simulink model "Model_TranslationEngine64"  (R2022b)
settings: Solver=FixedStepDiscrete  StartTime=0.0  StopTime=5  RelTol=1e-3  EnableMultiTasking=on
InitFcn:
  | % Initialize model
  | ModelSettings=BTConfig.GetModelSettings();
  | 
  | ModelSettings.Validate();
  | 
  | ModelInit;
  | 
  | 
  | % load library data
  | GainLibrary_data;
  | % Load saved values from partition process
  | CapturedConstMask.LoadMapFromFile(bdroot)
StartFcn:
  | % make sure all the simulated RTC requests are found
  | %RTC_SIM_OBJ.ValidateREQs();
undefined symbols (not defined in the file or in its folder): AA, BPLP, Column, NumHFRefBPF, NumHFRefLPF, NumMusicChannels, Row, VolumeMuteConfig
libraries: TuneVar x925, TOP x490, FeaturePath x111, CapturedConstLib x52
(part 3 of 34)

== system Model_TranslationEngine64/NEAR/Near1p1/DrProc ==
  FeaturePath : FeaturePath/FeaturePath  FeatureName=Dr_  IsGroup=off  GroupNumber=-1  IsModule=off  TriggerInit=[730 -106 845 1]
      settings: SourceProductName=Bose Talaria
  FsEQDr : Subsystem  mask(FsEQ){Config=Config.FsEqDr}
      mask prompts: Config "FsEqConfig"
      mask help:
      | This mask allows the setting of parameters for the FsEQ model.
      | Model parameters are set by a class instance in the base workspace.
      |
      | See 'Help' for details.
      mask init:
      | blkh=gcbh;
      | Config=BTConfig.Assert(blkh,Config);
      | 
      | Config.Validate();
      | Config.DoMaskInit(blkh);
      mask Help:
      | Defining model parameters:
      | The model parameters are set by the conents of an instance of FsEQClass.m.
      | 
      | To set model parameters:
      | 1-Create an instance of FsEQClass.m in the base workspace.
      | 2-In the model mask, set the 'Class instance' parameter to the name of the class instance in the base workspace.
      mask DialogControl ClassContainer Prompt: Name of class instance containing parameter settings
  HrEQDr : Subsystem  mask(HrEQ){Config=Config.HrEqDr}
      mask prompts: Config "HrEqConfig"
      mask help:
      | This mask allows the setting of parameters for the HrEQ model.
      | Model parameters are set by a class instance in the base workspace.
      |
      | See 'Help' for details.
      mask init:
      | blkh=gcbh;
      | Config=BTConfig.Assert(blkh,Config);
      | 
      | Config.Validate();
      | Config.DoMaskInit(blkh);
      mask Help:
      | Defining model parameters:
      | The model parameters are set by the conents of an instance of HrEQClass.m.
      | 
      | To set model parameters:
      | 1-Create an instance of HrEQClass.m in the base workspace.
      | 2-In the model mask, set the 'Class instance' parameter to the name of the class instance in the base workspace.
  RouterDr : Subsystem  mask(Bose Router){nInRouterMask=Config.NearRouterNumIn, nOutRouterMask=Config.NearRouterNumOut, outputMapDefaultRouterMask=Config.NearRouterMap}
      mask prompts: nInRouterMask "Number of input channels"; nOutRouterMask "Number of output channels"; outputMapDefaultRouterMask "Router output channel indices"
      mask help: This block allows the user to route X input channels to Y output channels. Enter a value of 0 to "zero out" the specific channel
      mask init:
      | blkh = gcbh;
      | % Copy discrete mask parameters into a classdef object
      | InnerLinkConfig = RouterConfig;
      | InnerLinkConfig.NumIn = nInRouterMask;
      | InnerLinkConfig.NumOut = nOutRouterMask;
      | InnerLinkConfig.DefaultOutputMap = outputMapDefaultRouterMask;
      mask Display: image('routerIcon.png');
  Upmixer1p1Dr : Subsystem  mask{Config=Config.Upmixer1p1Dr}
      mask prompts: Config "Upmixer1p1Config"
      mask init:
      | blkh=gcbh;
      | Config=BTConfig.Assert(blkh,Config);
      | % frontPeripheralChannelCount     = upmixer.front_peripheral_channel_count;
      | % headrest_count                  = upmixer.headrest_count;
      | % channels_per_headrest           = upmixer.channels_per_headrest;
      | Config.Validate();
      | Config.DoMaskInit(blkh);

== system Model_TranslationEngine64/NEAR/Near1p1/FrProc ==
  Subsystem : Subsystem

== system Model_TranslationEngine64/NEAR/Near1p1/LocRamper ==
  TuneTOP : Subsystem  mask(Talaria Trivial Tune TOP){TriggerInit=[-300 49 -55 141], TopName=RampDbPerSample, TuneName=RampDbPerSample, DataTypeOut=single, MaskValue=Config.DefaultRampDbPerSample, TunabilityNumber=1, MinValue=[], MaxValue=[], BankNumber=0, PreOverlay=false, PostOverlay=false, UseSameName=on}
      mask prompts: TriggerInit "Hidden: MoveFcn redraw"; TopName "Name:"; TuneName "Name of TuneVar:"; DataTypeOut "Data type:"; MaskValue "Default Value:"; TunabilityNumber "Tunability:"; MinValue "Min Value:"; MaxValue "Max Value:"; BankNumber "Target memory bank number:"; PreOverlay "Requires pre-overlay action:"; PostOverlay "Requires post-overlay action:"; UseSameName "Use same name for tune variable and TOP"
      mask help: The TuneTOP block encapsultes a Target Overlay Parameter, a Tune Variable, and a Trivial Translation between them.
      mask init:
      | [ok,activeTopPath,activeTunePath] = TuneTOP_Mask.Init(gcbh);
      settings: MoveFcn=TuneTOP_Mask.CB_TriggerInit(gcbh);
      mask Callback TriggerInit: TuneTOP_Mask.CB_TriggerInit(gcbh);
      mask TypeOptions TopName: TOP/TopName
      mask TypeOptions TuneName: Tune Variable/TuneName
      mask TypeOptions DataTypeOut: TOP/DataTypeOut
      mask TypeOptions MaskValue: Tune Variable/MaskValue
      mask TypeOptions TunabilityNumber: Tune Variable/TunabilityNumber
      mask Callback TunabilityNumber: TuneVarMask.CB_TunabilityNumber(gcbh);
      mask TypeOptions MinValue: Tune Variable/MinValue
      mask TypeOptions MaxValue: Tune Variable/MaxValue
      mask TypeOptions BankNumber: TOP/BankNumber
      mask TypeOptions PreOverlay: TOP/PreOverlay
      mask TypeOptions PostOverlay: TOP/PostOverlay
      mask Callback UseSameName: TuneTOP_Mask.CB_UseSameName(gcbh);
      mask DialogControl toolPanel Prompt: Tuning Tool Hints
      mask DialogControl DescriptionGroup Prompt: Description
      mask DialogControl EditDescription Prompt: Edit Description
      mask DialogControl EditDescription Callback: TuneTOP_Mask.CB_EditDescription(gcbh);
      mask DialogControl TunabilityText Prompt: Easy: Changes nearly every tuning.
      mask DialogControl AdvancedPanel Prompt: Advanced
      mask DialogControl ConvertToFullTranslation Prompt: Irreversible conversion to full translation
      mask DialogControl ConvertToFullTranslation Callback: TuneTOP_Mask.CB_ConvertToFullTranslation(gcbh);
      mask DialogControl ErrorContainer Prompt: Error Messages
      mask Display:
      | % retrieve icon definition
      | [path,w,h] = TuneTOP_Mask.Icon();
      | 
      | % retrieve the block's pixel size
      | pos = get(gcbh,'position');
      | bw = pos(3) - pos(1);
      | bh = pos(4) - pos(2);
      | 
      | % draw centered icon
      | xAdj = bw/2 - w/2 + 5;
      | yAdj = bh/2 - h/2 + 4;
      | for i=1:length(path)
      | 	patch(path(i).x+xAdj, path(i).y+yAdj, path(i).rgb);
      | end
      | 
      | % show the top name or an X
      | if (exist('ok','var') && ok)
      | 	text(bw*0.5, bh*0.2, activeTopPath, 'horizontalAlignment', 'center');
      | 	patch(0,0,[1 1 1]);
      | 	patch(bw,bh,[1 1 1]);
      | else
      | 	tx=bw*0.03;
      | 	ty=bh*0.03;
      | 	patch([0 tx bw bw-tx], [ty 0 bh-ty bh], [1 0 0]);
      | 	patch([0 bw-tx bw tx], [bh-ty 0 ty bh], [1 0 0]);
      | end

== system Model_TranslationEngine64/NEAR/Near1p1/NearBandSplit ==
  HighpassFilter : Subsystem

== system Model_TranslationEngine64/NEAR/Near1p1/VolumeMute ==
  AnnouncementLevelDetector : Subsystem  mask(Level Detector for AudioPilot, Dyanmic EQ, Fan and Boost-on-Demand){vm=VolumeMuteConfig, DefaultFlag=off, Config=Config.AnnouncementLevelDetector}
      mask prompts: vm "Vm Class Instance"; DefaultFlag "Use Default Configuration Only"; Config "AnnouncementLevelDetectorConfig"
      mask help: This block performs level detection, separately and independently, for various features. These include AudioPilot, Dynamic Equalization, Amplifier Fan Control, and Boost on Demand. The block is designed to accept as input the entertainment audio channels before volume control was applied. The volume setting, in linear, forms a different input.
      mask init:
      | blkh=gcbh;
      | Config=BTConfig.Assert(blkh,Config);
      | % if DefaultFlag
      | %     LD = struct();
      | % end
      | %[LD, SampleRate, FrameRate, MaxMusicDelay] ...
      | %    = AnnouncementLevelDetectionMask.Initialize(gcbh,LD,vm);
      | Config.Validate();
      | Config.DoMaskInit(blkh);
      mask Callback DefaultFlag: % AnnouncementLevelDetectionMask.DefaultFlagCallBack(gcbh);
  VolMuteCh1 : Subsystem
  VolMuteCh2 : Subsystem
  VolMuteCh3 : Subsystem
  VolMuteCh4 : Subsystem

== system Model_TranslationEngine64/PostProcess/PostProcess/Limiter ==
  Limiter : Subsystem  mask(Blocklib Limiter){Config=Config.Limiter, FeatureName=Limiter}
      mask prompts: Config "LimiterConfig"; FeatureName "Feature path name:"
      mask init:
      | blkh=gcbh;
      | Config=BTConfig.Assert(blkh,Config);
      | 
      | Config.Validate();
      | BTConfig.InitSetFeatureIfPresent(blkh,'FeatureName');
      mask Callback Config: BTConfig.CallbackHideIfPresent(gcbh,{'FeatureName'});
      mask TypeOptions FeatureName: FeaturePath/FeatureName
      mask Display:
      | [path,w,h] = IconLimiterMask();
      | 
      | % work in pixels since the icon does not scale
      | pos = get(gcbh,'position');
      | bw = pos(3) - pos(1);
      | bh = pos(4) - pos(2);
      | 
      | % Draw centered icon
      | xAdj = bw/2 - w/2;
      | yAdj = bh/2 - h/2 + 4;
      | for i=1:length(path)
      |     if (path(i).rgb(1) >= 0)
      |         patch(path(i).x+xAdj, path(i).y+yAdj, path(i).rgb);
      |     end
      |     if (path(i).stroke(1) >= 0)
      |         plot(path(i).x+xAdj, path(i).y+yAdj);
      |     end
      | end
      | 
      | % Display some text
      | text(bw/2, 4,FeatureName, ...
      |     'horizontalAlignment','center', ...
      |     'VerticalAlignment','bottom');

== system Model_TranslationEngine64/PostProcess/PostProcess/Mute ==
  Mute : Subsystem  mask(Blocklib Mute){Config=Config.Mute, FeatureName=Mute}
      mask prompts: Config "MuteConfig"; FeatureName "Feature path name:"
      mask help: This block offers a simple mute feature using rgainy block. Set initial mute state for system cold start and a feature path name as desired. There are no tunable components, but runtime control is included.
      mask init:
      | blkh=gcbh;
      | Config=BTConfig.Assert(blkh,Config);
      | BTConfig.InitSetFeatureIfPresent(blkh,'FeatureName');
      | Config.Validate();
      mask Help:
      | This block offers a simple mute feature using rgainy block. The initial mute status of the block can be set through the mask.
      | 
      | RTC CONTROL:
      | Run time control is available to dynamically mute the audio. The mute status can be provided ('1' to mute audio), along with a ramp time and rate (rate gets precedence).
      | RTC_SIM_OBJ.AddREQ( 'MuteSet', 0.6, [0005,  <mute_status>, <ramp_db_per_second>, <ramp_time>]);
      | E.g., RTC_SIM_OBJ.AddREQ( 'MuteSet', 0.7, [0002, 1, 0, 50]);
      mask Callback Config: BTConfig.CallbackHideIfPresent(gcbh,{'FeatureName'});
      mask TypeOptions FeatureName: MuteControl/FeatureName
      mask Display:
      | [path,w,h] = IconMuteMask();
      | 
      | % work in pixels since the icon does not scale
      | pos = get(gcbh,'position');
      | bw = pos(3) - pos(1);
      | bh = pos(4) - pos(2);
      | 
      | % Draw centered icon
      | xAdj = bw/2 - w/2;
      | yAdj = bh/2 - h/2;
      | for i=1:length(path)
      |     if (path(i).rgb(1) >= 0)
      |         patch(path(i).x+xAdj, path(i).y+yAdj, path(i).rgb);
      |     end
      |     if (path(i).stroke(1) >= 0)
      |         plot(path(i).x+xAdj, path(i).y+yAdj);
      |     end
      | end
      | 
      | % Display some text
      | text(bw/2, 2,FeatureName, ...
      |     'horizontalAlignment','center', ...
      |     'VerticalAlignment','bottom');

== system Model_TranslationEngine64/PostProcess/PostProcess/PostLimiterEQ ==
  PoolIirTunableWithReset : Subsystem  mask(Bose Pool IIR Tunable){FeatureName=PostLimiterEq, Config=Config.PostLimiterEq}
      mask prompts: FeatureName "Filter name/purpose"; Config "PoolIirTunableWithResetConfig"
      mask help:
      | Pool IIR Tunable is a configurable multi-channel IIR filter that supports one or more channels. This block offers flexibility of tuning the number of stages and coefficients. Different filter coefficients and number of stages (biquads) can be used for each channel filter. The Pool IIR Tunable block supports different implementations, which could be configured at build-time:
      |
      | (i)   Generic: IIR filter code not optimized for any processor
      | (ii)  SharcCore: IIR filters executing on core (uses pooliir.asm CRL)
      | (iii) SharcGulAccel: IIR filters executing on IIR hardware accelerator, offloading MIPS usage from core
      | (iv) SharcGxpAccel: IIR filters take advantage of additional accelerators available on GXP processor
      | (v)  Hexagon: TBD
      |
      | NOTE: When using Pool IIR for Sharc-plus based processors, the codeWorkMemory buffer and input buffer should always be mapped to L1 memory to optimize MIPS utilization and avoid audio artifacts.
      |
      | For more information, please see 'Help'.
      mask init:
      | blkh=gcbh;
      | Config=BTConfig.Assert(blkh,Config);
      | 
      | BTConfig.InitSetFeatureIfPresent(blkh,'FeatureName');
      | Config.Validate();
      | Config.DoMaskInit(blkh);
      mask Help:
      | <b>Input signals: </b>
      | AudioIn: input channels [frame size x number of channels]
      | ResetTrigger: trigger to reset internal state buffer (usually preferred as a post RMDL step)
      | 
      | <b>Output signals: </b>
      | AudioOut: output channels [frame size x number of channels]
      | 
      | <b>Mask parameters: </b>
      | PoolIirTunableWithResetConfig
      | Filter name/purpose
      mask TypeOptions FeatureName: FeaturePath/FeatureName
      mask Callback Config: BTConfig.CallbackHideIfPresent(gcbh,{'FeatureName'});
      mask Display: DrawPoolIirIcon;

== system Model_TranslationEngine64/PostProcess/PostProcess/Soft Clipper ==
  SoftClipper : Subsystem  mask(Blocklib SoftClipper){Config=Config.SoftClipper, FeatureName=SoftClipper}
      mask prompts: Config "SoftClipperConfig"; FeatureName "Feature path name:"
      mask init:
      | blkh=gcbh;
      | Config=BTConfig.Assert(blkh,Config);
      | 
      | Config.Validate();
      | BTConfig.InitSetFeatureIfPresent(blkh,'FeatureName');
      mask Callback Config: BTConfig.CallbackHideIfPresent(gcbh,{'FeatureName'});
      mask TypeOptions FeatureName: FeaturePath/FeatureName
      mask Display:
      | [path,w,h] = IconSoftclipperMask();
      | 
      | % work in pixels since the icon does not scale
      | pos = get(gcbh,'position');
      | bw = pos(3) - pos(1);
      | bh = pos(4) - pos(2);
      | 
      | % Draw centered icon
      | xAdj = bw/2 - w/2;
      | yAdj = bh/2 - h/2 + 4;
      | for i=1:length(path)
      |     if (path(i).rgb(1) >= 0)
      |         patch(path(i).x+xAdj, path(i).y+yAdj, path(i).rgb);
      |     end
      |     if (path(i).stroke(1) >= 0)
      |         plot(path(i).x+xAdj, path(i).y+yAdj);
      |     end
      | end
      | 
      | % Display some text
      | text(bw/2, 4,FeatureName, ...
      |     'horizontalAlignment','center', ...
      |     'VerticalAlignment','bottom');

== system Model_TranslationEngine64/TestRouter/ASDRouter/InnerLink ==
  AuxChannel_with_MATLAB_function : Subsystem
  FeaturePath : FeaturePath/FeaturePath  FeatureName=ASDRouter  IsGroup=off  GroupNumber=-1  IsModule=off  TriggerInit=[-50 -126 65 -19]
      settings: SourceProductName=Bose Talaria
  MainChannelSystem : Subsystem

== system Model_TranslationEngine64/ModelPreAmp/DecRate/AudioPilot35/Audiopilot_3_5 ==
  ConfigurationRtcInputs : Subsystem
  FeaturePath : FeaturePath/FeaturePath  FeatureName=Audiopilot  IsGroup=off  GroupNumber=-1  IsModule=off  TriggerInit=[1175 264 1290 371]
      settings: SourceProductName=Bose Talaria
  GainApplication : Subsystem  mask(AudioPilot - Loudness Gain Application){NumInputChannels=NumMusicChannels, Config=Config.GainApp}
      mask prompts: NumInputChannels "Number of Input Channels"; Config "GainApplicationConfig"
      mask help: This block implements the necessary compensation to the audio stream for AudioPilot and Dynamic EQ.
      mask init:
      | blkh = gcbh;
      | 
      | Config = BTConfig.Assert(blkh,Config);
      | Config.Validate();
      | 
      | SampleRate = Config.SampleRateHz;
      | FrameSize = Config.FrameSize;
      | oneFrame = ones(FrameSize,1);
      | MaxAlignDelaySamples = Config.MidrangeLpfMaxAlignDelaySamples;
      mask Help:
      | This block implements the necessary compensation to the audio stream for AudioPilot and Dynamic EQ.
      | 
      | Arguments for this block:
      | 
      | Number of Music Channels
      | This is the number of input audio channels to be processed, typically 2 for stereo or 6 for surround.
      | 
      | Build Time Configuration
      | The block can be configured using an object of class, GainApplicationConfig.
      mask DialogControl DTC Prompt: Design Time Configuration
      mask DialogControl BTC Prompt: Build Time Configuration
  GainCalculation : Subsystem  mask(AudioPilot - Gain Calculation){Config=Config.GainCalc}
      mask prompts: Config "GainCalculationConfig"
      mask help: This block implements the gain calculations for AudioPilot and Dynamic EQ.
      mask init:
      | blkh = gcbh;
      | 
      | Config = BTConfig.Assert(blkh,Config);
      | Config.Validate();
      | 
      | SampleRate = Config.SampleRateHz;
      | FrameSize = Config.FrameSize;
      | FrameRate = Config.FrameRateHz;
      | 
      | % Configure RTC responses            
      | GainCalculationMask.ConfigureRtcResponses(blkh,...
      |                 Config.EnableRtcResponse)
      mask Help:
      | This block implements the gain calculations for AudioPilot and Dynamic EQ.
      | 
      | Arguments for this block:
      | 
      | Configuration
      | The block can be configured using an object of class, GainCalculationConfig.
      mask DialogControl BTC Prompt: Build Time Configuration
      mask DialogControl Config Tooltip: The configuration has to be an object of the class, GainCalculationConfig.
  NoiseEstimationVariant : Subsystem  Variant=on  VariantControlMode=label  LabelModeActiveChoice=Regular  PropagateVariantConditions=on

== system Model_TranslationEngine64/ModelPreAmp/DecRate/AudioPilot35/EntertainmentLevelDetection ==
  AudiopilotLevelDetect : Subsystem
  DyneqLevelDetect : Subsystem
  PreProcessing : Subsystem

== system Model_TranslationEngine64/ModelPreAmp/DecRate/AudioPilot35/Volume ==
  FeaturePath : FeaturePath/FeaturePath  FeatureName=VolumeCfg  IsGroup=off  GroupNumber=-1  IsModule=off  TriggerInit=[640 269 755 376]
      settings: SourceProductName=Bose Talaria
  Index2DbTable : Subsystem  mask(Blocklib Index2DbTable){Config=Config}
      mask prompts: Config "Index2DbTableConfig"
      mask help: This block contains overlay tuning data for an index-to-dB lookup table. Provide the maximum number of points in the table as a build-time variable. The TuneVar is variable size, but must define at least two points (i.e. two rows, or four values).
      mask init:
      | blkh=gcbh;
      | Config=BTConfig.Assert(blkh,Config);
      | 
      | Config.Validate();
      mask Help:
      | This block contains overlay tuning data which defines an index-to-dB lookup table.
      | Each row of the tuning data contains an index and a dB value.
      | 
      | Tuning data
      | ---------------
      |    tune index: normalized value between 0 and 1
      |    tune value: dB value such as 0 (aka linear "1") or -100 (aka "very quiet")
      | 
      | Inports
      | ----------
      |    trigger: function call trigger that invokes the lookup from inport index to output dB
      |    index: an 8-bit integer index between [0:255] corresponding to the tuning index range [0:1]
      | 
      | Outport
      | -----------
      |    The resulting dB value looked up in the tuned table by using the inbound index
  TuneVarRampTimeMs : Subsystem  mask(Talaria Trivial Tune TOP){TriggerInit=[825 324 910 356], TopName=RampTime, TuneName=RampTime, DataTypeOut=single, MaskValue=100, TunabilityNumber=1, MinValue=[], MaxValue=[], BankNumber=0, PreOverlay=false, PostOverlay=false, UseSameName=on}
      mask prompts: TriggerInit "Hidden: MoveFcn redraw"; TopName "Name:"; TuneName "Name of TuneVar:"; DataTypeOut "Data type:"; MaskValue "Default Value:"; TunabilityNumber "Tunability:"; MinValue "Min Value:"; MaxValue "Max Value:"; BankNumber "Target memory bank number:"; PreOverlay "Requires pre-overlay action:"; PostOverlay "Requires post-overlay action:"; UseSameName "Use same name for tune variable and TOP"
      mask help: The TuneTOP block encapsultes a Target Overlay Parameter, a Tune Variable, and a Trivial Translation between them.
      mask init:
      | [ok,activeTopPath,activeTunePath] = TuneTOP_Mask.Init(gcbh);
      settings: MoveFcn=TuneTOP_Mask.CB_TriggerInit(gcbh);
      mask Callback TriggerInit: TuneTOP_Mask.CB_TriggerInit(gcbh);
      mask TypeOptions TopName: TOP/TopName
      mask TypeOptions TuneName: Tune Variable/TuneName
      mask TypeOptions DataTypeOut: TOP/DataTypeOut
      mask TypeOptions MaskValue: Tune Variable/MaskValue
      mask TypeOptions TunabilityNumber: Tune Variable/TunabilityNumber
      mask Callback TunabilityNumber: TuneVarMask.CB_TunabilityNumber(gcbh);
      mask TypeOptions MinValue: Tune Variable/MinValue
      mask TypeOptions MaxValue: Tune Variable/MaxValue
      mask TypeOptions BankNumber: TOP/BankNumber
      mask TypeOptions PreOverlay: TOP/PreOverlay
      mask TypeOptions PostOverlay: TOP/PostOverlay
      mask Callback UseSameName: TuneTOP_Mask.CB_UseSameName(gcbh);
      mask DialogControl toolPanel Prompt: Tuning Tool Hints
      mask DialogControl DescriptionGroup Prompt: Description
      mask DialogControl EditDescription Prompt: Edit Description
      mask DialogControl EditDescription Callback: TuneTOP_Mask.CB_EditDescription(gcbh);
      mask DialogControl TunabilityText Prompt: Easy: Changes nearly every tuning.
      mask DialogControl AdvancedPanel Prompt: Advanced
      mask DialogControl ConvertToFullTranslation Prompt: Irreversible conversion to full translation
      mask DialogControl ConvertToFullTranslation Callback: TuneTOP_Mask.CB_ConvertToFullTranslation(gcbh);
      mask DialogControl ErrorContainer Prompt: Error Messages
      mask Display:
      | % retrieve icon definition
      | [path,w,h] = TuneTOP_Mask.Icon();
      | 
      | % retrieve the block's pixel size
      | pos = get(gcbh,'position');
      | bw = pos(3) - pos(1);
      | bh = pos(4) - pos(2);
      | 
      | % draw centered icon
      | xAdj = bw/2 - w/2 + 5;
      | yAdj = bh/2 - h/2 + 4;
      | for i=1:length(path)
      | 	patch(path(i).x+xAdj, path(i).y+yAdj, path(i).rgb);
      | end
      | 
      | % show the top name or an X
      | if (exist('ok','var') && ok)
      | 	text(bw*0.5, bh*0.2, activeTopPath, 'horizontalAlignment', 'center');
      | 	patch(0,0,[1 1 1]);
      | 	patch(bw,bh,[1 1 1]);
      | else
      | 	tx=bw*0.03;
      | 	ty=bh*0.03;
      | 	patch([0 tx bw bw-tx], [ty 0 bh-ty bh], [1 0 0]);
      | 	patch([0 bw-tx bw tx], [bh-ty 0 ty bh], [1 0 0]);
      | end

== system Model_TranslationEngine64/ModelPreAmp/DecRate/Medusa5H1/Balance ==
  Balance : Subsystem  mask(Blocklib Balance){FeatureName=Balance_Cfg, Config=Config.Balance_Cfg}
      mask prompts: FeatureName "Feature path name:"; Config "BalanceConfig"
      mask help:
      | This Balance block allows for runtime control of balancing between left and right speakers/content. Based on a gain index which comes in through a control message, channel gains for 4 different content types are computed: Left, Right, Center, and Mono.
      |
      | For the Channel to Ramper Map, enter any of the following values:
      | 1 - left channel
      | 2 - right channel
      | 3 - center channel
      | 4 - mono channel
      | -1 - unused channel (will esentially be muted)
      |
      | Enable Silent Extreme if the desired outcome when accepting an index of 0 (hard left) or 255 (hard right) should completely mute the opposing channel.
      |
      | If Silent Extreme Mutes Bass is enabled, then all mono channels will be muted, when Silent Extreme is activated.
      |
      | If this block is being used in conjunction with a stand-alone Sleeping Beauty block, disable the two Silent Extreme options.
      mask init:
      | blkh=gcbh;
      | Config=BTConfig.Assert(blkh,Config);
      | 
      | BTConfig.InitSetFeatureIfPresent(blkh,'FeatureName');
      | Config.Validate();
      | 
      | % Mask init code
      | BalanceMask.Init(blkh);
      | 
      | % Flatten config for MFBs
      | MaskNumRampers = Config.NumRampers;
      | MaskBlockH = blkh;
      | % Set boundary conditions (are these supposed to be BTC?)
      | rampRateBounds = [5,50000];
      | rampTimeBounds = [1,3000];
      mask Help:
      | The Balance block includes runtime control support for adjusting the balance dynamically.
      | - Channels may to be assigned to one of 4 possible rampers. Each channel needs to be assigned to a valid ramper (i.e. 1 - 4, or -1 for unused).
      | - The Index offset determines the index which corresponds to the balance being in the center position (typically 128).
      | - 'Enable silent extreme' mutes the speakers of the group whose gains are being 'cut' when at extreme indices.
      | - 'Disable boost' determines whether a boost is required or not. If selected, the maximum boost will be '1' on the linear scale ('0' in dB), otherwise he boost is calculated based on the curve (typically a maximum of 3 dB).
      | 
      | Control messages can be sent through the RTC block. The block is configured to accept a ramp time or rate (the rate has precedence) and an index which determines the gains for each channel group.
      | E.g., RTC_SIM_OBJ.AddREQ( 'BalanceSet', 0.1, [0001, <balance_index>, <ramp_db_per_second>, <ramp_milliseconds>, <subwoofer_index>, <surround_volume_index>]);
      | E.g., RTC_SIM_OBJ.AddREQ( 'BalanceSet', 0.1, [0001, 255, 0, 50, 128, 192]);
      mask TypeOptions FeatureName: FeaturePath/FeatureName
      mask Callback Config: BTConfig.CallbackHideIfPresent(gcbh,{'FeatureName'});
      mask Display:
      | [path,w,h] = IconBalanceMask();
      | 
      | % work in pixels since the icon does not scale
      | pos = get(gcbh,'position');
      | bw = pos(3) - pos(1);
      | bh = pos(4) - pos(2);
      | 
      | % Draw centered icon
      | xAdj = bw/2 - w/2;
      | yAdj = bh/2 - h/2;
      | for i=1:length(path)
      |     if (path(i).rgb(1) >= 0)
      |         patch(path(i).x+xAdj, path(i).y+yAdj, path(i).rgb);
      |     end
      |     if (path(i).stroke(1) >= 0)
      |         plot(path(i).x+xAdj, path(i).y+yAdj);
      |     end
      | end
      | 
      | % place feature name text
      | text(bw*0.5, 0, [FeatureName '\n\n'], 'horizontalAlignment', 'center');

== system Model_TranslationEngine64/ModelPreAmp/DecRate/Medusa5H1/MedusaHoligram ==
  FeaturePath : FeaturePath/FeaturePath  FeatureName=Medusa  IsGroup=off  GroupNumber=-1  IsModule=off  TriggerInit=[90 69 205 176]
      settings: SourceProductName=Bose Talaria
  Medusa5H1 Part 1 : Subsystem  TreatAsAtomicUnit=on
      settings: RTWSystemCode=Nonreusable function
  Medusa5H1 Part 2 : Subsystem  TreatAsAtomicUnit=on
      settings: RTWSystemCode=Nonreusable function
  Medusa5H1 Part 3 : Subsystem  TreatAsAtomicUnit=on
      settings: RTWSystemCode=Nonreusable function  FunctionWithSeparateData=on
  Medusa5H1 Part 4 : Subsystem  TreatAsAtomicUnit=on  RTWFcnName=MedusaHoligram  RTWFileName=MedusaHoligram
      settings: RTWSystemCode=Nonreusable function  FunctionWithSeparateData=on
  Medusa5H1 Part 6 : Subsystem  TreatAsAtomicUnit=on
      settings: RTWSystemCode=Nonreusable function  FunctionWithSeparateData=on

== system Model_TranslationEngine64/ModelPreAmp/DecRate/Medusa5H1/MedusaPostHoligram ==
  MedusaPostHoligram : Subsystem  TreatAsAtomicUnit=on  mask{config=Config.MedusaConfig}
      mask prompts: config "Config struct name:"
      settings: RTWSystemCode=Nonreusable function  RTWFcnNameOpts=Use subsystem name  RTWFileNameOpts=Use subsystem name  FunctionWithSeparateData=on

== system Model_TranslationEngine64/ModelPreAmp/DecRate/Medusa5H1/NearWiggleFilters ==
  NEAR : Subsystem  Variant=on  VariantControl=Variant1

== system Model_TranslationEngine64/ModelPreAmp/DecRate/Medusa5H1/SleepingBeauty ==
  SleepingBeauty : Subsystem  Variant=on  VariantControl=Choice

== system Model_TranslationEngine64/ModelPreAmp/DecRate/Medusa5H1/VLS ==
  Crosstalk Cancellation : Subsystem  mask{configStruct=configStruct.XtalkCancellationConfig}
      mask prompts: configStruct "Config struct name:"
      mask init:
      | IIR = configStruct.IIR;
      mask Display:
      | port_label('input', 1, sprintf('Le_D, Re_D,\nLe_P, Re_P'));
      | port_label('output', 1, 'SpkrOut');
  FeaturePath : FeaturePath/FeaturePath  FeatureName=VLS  IsGroup=off  GroupNumber=-1  IsModule=off  TriggerInit=[1295 -226 1410 -119]
      settings: SourceProductName=Bose Talaria
  VLS Generation - D : Subsystem  mask{configStruct=configStruct.VLSGenDConfig, FeatureName=GenerationDrv}
      mask prompts: configStruct "Config struct name:"; FeatureName "Feature path name:"
      mask init:
      | % Get block parameters from configStruct
      | variantFIR = configStruct.variantFIR;
      | frameSize = configStruct.frameSize;
      | numFilters = configStruct.numFilters;
      | maxTotalFirLength = configStruct.maxTotalFirLength;
      | 
      | % Get block default values
      | firCoeffsDefault = configStruct.firCoeffsDefault;
      | firLengthsDefault = configStruct.firLengthsDefault;
      | 
      | % Set implementation type for FIR
      | % firBlockPath = MaskUtil.SubBlockName(gcbh, 'FIR');
      | % firBlockHandle = getSimulinkBlockHandle(firBlockPath);
      | % if -1 ~= firBlockHandle
      | %     set_param(firBlockHandle, 'variantSelect', variantFIR);
      | %     if variantFIR == 1 % Set two extras block params for Accel implementation
      | %         set_param(firBlockHandle, 'numIn', num2str(4));
      | %         set_param(firBlockHandle, 'frameSize', num2str(frameSize));
      | %     end
      | % end
      mask TypeOptions FeatureName: FeaturePath/FeatureName
  VLS Generation - P : Subsystem  mask{configStruct=configStruct.VLSGenPConfig, FeatureName=GenerationPax}
      mask prompts: configStruct "Config struct name:"; FeatureName "Feature path name:"
      mask init: same as Model_TranslationEngine64/ModelPreAmp/DecRate/Medusa5H1/VLS/VLS Generation - D
      mask TypeOptions FeatureName: FeaturePath/FeatureName

== system Model_TranslationEngine64/ModelPreAmp/PreAmpPart1/Bass/TuneVarOffset ==
  TOP : TOP/TOP  TriggerInit=[440 20 585 80]  TopName=Offset  DataTypeOut=single  BankNumber=BankNumber  PreOverlay=PreOverlay  PostOverlay=PostOverlay  Role=Automatic
      settings: SourceProductName=Bose Talaria
  TrivialTranslation : TuneVar/TrivialTranslation  TriggerInit=[300 28 350 72]
      settings: SourceProductName=Bose Talaria
  Tune Variable : TuneVar/TuneVar  TuneName=Offset  SpecifyMaxSize=off  VariableDim=1 (Row)  MaxSize=[1 1]  TunabilityNumber=1  MinValue=MinValue  MaxValue=MaxValue  TriggerInit=[20 25 190 75]  MaskValue=MaskValue
      settings: SourceProductName=Bose Talaria
  wires:
  Tune Variable/1 -> TrivialTranslation/1  "Offset"
  TrivialTranslation/1 -> TOP/1

== system Model_TranslationEngine64/ModelPreAmp/PreAmpPart1/Bass/TuneVarRampTime ==
  TOP : TOP/TOP  TriggerInit=[440 20 585 80]  TopName=ramptime  DataTypeOut=single  BankNumber=BankNumber  PreOverlay=PreOverlay  PostOverlay=PostOverlay  Role=Automatic
      settings: SourceProductName=Bose Talaria
  TrivialTranslation : TuneVar/TrivialTranslation  TriggerInit=[300 28 350 72]
      settings: SourceProductName=Bose Talaria
  Tune Variable : TuneVar/TuneVar  TuneName=ramptime  SpecifyMaxSize=off  VariableDim=1 (Row)  MaxSize=[1 1]  TunabilityNumber=1  MinValue=MinValue  MaxValue=MaxValue  TriggerInit=[20 25 190 75]  MaskValue=MaskValue
      settings: SourceProductName=Bose Talaria
  wires:
  Tune Variable/1 -> TrivialTranslation/1  "ramptime"
  TrivialTranslation/1 -> TOP/1

== system Model_TranslationEngine64/ModelPreAmp/PreAmpPart1/Bass/TuneVarScale ==
  TOP : TOP/TOP  TriggerInit=[440 20 585 80]  TopName=Scale  DataTypeOut=single  BankNumber=BankNumber  PreOverlay=PreOverlay  PostOverlay=PostOverlay  Role=Automatic
      settings: SourceProductName=Bose Talaria
  TrivialTranslation : TuneVar/TrivialTranslation  TriggerInit=[300 28 350 72]
      settings: SourceProductName=Bose Talaria
  Tune Variable : TuneVar/TuneVar  TuneName=Scale  SpecifyMaxSize=off  VariableDim=1 (Row)  MaxSize=[1 1]  TunabilityNumber=1  MinValue=MinValue  MaxValue=MaxValue  TriggerInit=[20 25 190 75]  MaskValue=MaskValue
      settings: SourceProductName=Bose Talaria
  wires:
  Tune Variable/1 -> TrivialTranslation/1  "Scale"
  TrivialTranslation/1 -> TOP/1

== system Model_TranslationEngine64/ModelPreAmp/PreAmpPart1/Midrange/TuneVarOffset ==
  TOP : TOP/TOP  TriggerInit=[440 20 585 80]  TopName=Offset  DataTypeOut=single  BankNumber=BankNumber  PreOverlay=PreOverlay  PostOverlay=PostOverlay  Role=Automatic
      settings: SourceProductName=Bose Talaria
  TrivialTranslation : TuneVar/TrivialTranslation  TriggerInit=[300 28 350 72]
      settings: SourceProductName=Bose Talaria
  Tune Variable : TuneVar/TuneVar  TuneName=Offset  SpecifyMaxSize=off  VariableDim=1 (Row)  MaxSize=[1 1]  TunabilityNumber=1  MinValue=MinValue  MaxValue=MaxValue  TriggerInit=[20 25 190 75]  MaskValue=MaskValue
      settings: SourceProductName=Bose Talaria
  wires:
  Tune Variable/1 -> TrivialTranslation/1  "Offset"
  TrivialTranslation/1 -> TOP/1

== system Model_TranslationEngine64/ModelPreAmp/PreAmpPart1/Midrange/TuneVarRampTime ==
  TOP : TOP/TOP  TriggerInit=[440 20 585 80]  TopName=RampTime  DataTypeOut=single  BankNumber=BankNumber  PreOverlay=PreOverlay  PostOverlay=PostOverlay  Role=Automatic
      settings: SourceProductName=Bose Talaria
  TrivialTranslation : TuneVar/TrivialTranslation  TriggerInit=[300 28 350 72]
      settings: SourceProductName=Bose Talaria
  Tune Variable : TuneVar/TuneVar  TuneName=RampTime  SpecifyMaxSize=off  VariableDim=1 (Row)  MaxSize=[1 1]  TunabilityNumber=1  MinValue=MinValue  MaxValue=MaxValue  TriggerInit=[20 25 190 75]  MaskValue=MaskValue
      settings: SourceProductName=Bose Talaria
  wires:
  Tune Variable/1 -> TrivialTranslation/1  "RampTime"
  TrivialTranslation/1 -> TOP/1

== system Model_TranslationEngine64/ModelPreAmp/PreAmpPart1/Midrange/TuneVarScale ==
  TOP : TOP/TOP  TriggerInit=[440 20 585 80]  TopName=Scale  DataTypeOut=single  BankNumber=BankNumber  PreOverlay=PreOverlay  PostOverlay=PostOverlay  Role=Automatic
      settings: SourceProductName=Bose Talaria
  TrivialTranslation : TuneVar/TrivialTranslation  TriggerInit=[300 28 350 72]
      settings: SourceProductName=Bose Talaria
  Tune Variable : TuneVar/TuneVar  TuneName=Scale  SpecifyMaxSize=off  VariableDim=1 (Row)  MaxSize=[1 1]  TunabilityNumber=1  MinValue=MinValue  MaxValue=MaxValue  TriggerInit=[20 25 190 75]  MaskValue=MaskValue
      settings: SourceProductName=Bose Talaria
  wires:
  Tune Variable/1 -> TrivialTranslation/1  "Scale"
  TrivialTranslation/1 -> TOP/1

== system Model_TranslationEngine64/ModelPreAmp/PreAmpPart1/NEARPreAmp/FixedAttenuator ==
  "Attenuation " : Subsystem

== system Model_TranslationEngine64/ModelPreAmp/PreAmpPart1/NEARPreAmp/Monoizer ==
  Monoizer : Subsystem  Variant=on  VariantControl=Choice

== system Model_TranslationEngine64/ModelPreAmp/PreAmpPart1/NEARPreAmp/MusicLimiter ==
  annPredTuneTOP : Subsystem
  limiter : Subsystem
      mask DialogControl Container3 Prompt: Parameter Set
      mask Display:
      | [path,w,h] = IconLimiterMask();
      | 
      | % work in pixels since the icon does not scale
      | pos = get(gcbh,'position');
      | bw = pos(3) - pos(1);
      | bh = pos(4) - pos(2);
      | 
      | % Draw centered icon
      | xAdj = bw/2 - w/2;
      | yAdj = bh/2 - h/2 + 4;
      | for i=1:length(path)
      |     if (path(i).rgb(1) >= 0)
      |         patch(path(i).x+xAdj, path(i).y+yAdj, path(i).rgb);
      |     end
      |     if (path(i).stroke(1) >= 0)
      |         plot(path(i).x+xAdj, path(i).y+yAdj);
      |     end
      | end
      | 
      | % Anchor the corners of the coordinate system
      | patch(0,0,[1 1 1]);
      | patch(bw,bh,[1 1 1]);
      | 
      | % Display some text
      | text(bw/2, 4,'Limiter', ...
      |     'horizontalAlignment','center', ...
      |     'VerticalAlignment','bottom');
  offsetTuneTOP : Subsystem
  upperThresholdTuneTOP : Subsystem

== system Model_TranslationEngine64/ModelPreAmp/PreAmpPart1/Treble/TuneVarOffset ==
  TOP : TOP/TOP  TriggerInit=[440 20 585 80]  TopName=Offset  DataTypeOut=single  BankNumber=BankNumber  PreOverlay=PreOverlay  PostOverlay=PostOverlay  Role=Automatic
      settings: SourceProductName=Bose Talaria
  TrivialTranslation : TuneVar/TrivialTranslation  TriggerInit=[300 28 350 72]
      settings: SourceProductName=Bose Talaria
  Tune Variable : TuneVar/TuneVar  TuneName=Offset  SpecifyMaxSize=off  VariableDim=1 (Row)  MaxSize=[1 1]  TunabilityNumber=1  MinValue=MinValue  MaxValue=MaxValue  TriggerInit=[20 25 190 75]  MaskValue=MaskValue
      settings: SourceProductName=Bose Talaria
  wires:
  Tune Variable/1 -> TrivialTranslation/1  "Offset"
  TrivialTranslation/1 -> TOP/1

== system Model_TranslationEngine64/ModelPreAmp/PreAmpPart1/Treble/TuneVarRampTime ==
  TOP : TOP/TOP  TriggerInit=[440 20 585 80]  TopName=ramptime  DataTypeOut=single  BankNumber=BankNumber  PreOverlay=PreOverlay  PostOverlay=PostOverlay  Role=Automatic
      settings: SourceProductName=Bose Talaria
  TrivialTranslation : TuneVar/TrivialTranslation  TriggerInit=[300 28 350 72]
      settings: SourceProductName=Bose Talaria
  Tune Variable : TuneVar/TuneVar  TuneName=ramptime  SpecifyMaxSize=off  VariableDim=1 (Row)  MaxSize=[1 1]  TunabilityNumber=1  MinValue=MinValue  MaxValue=MaxValue  TriggerInit=[20 25 190 75]  MaskValue=MaskValue
      settings: SourceProductName=Bose Talaria
  wires:
  Tune Variable/1 -> TrivialTranslation/1  "ramptime"
  TrivialTranslation/1 -> TOP/1

== system Model_TranslationEngine64/ModelPreAmp/PreAmpPart1/Treble/TuneVarScale ==
  TOP : TOP/TOP  TriggerInit=[440 20 585 80]  TopName=Scale  DataTypeOut=single  BankNumber=BankNumber  PreOverlay=PreOverlay  PostOverlay=PostOverlay  Role=Automatic
      settings: SourceProductName=Bose Talaria
  TrivialTranslation : TuneVar/TrivialTranslation  TriggerInit=[300 28 350 72]
      settings: SourceProductName=Bose Talaria
  Tune Variable : TuneVar/TuneVar  TuneName=Scale  SpecifyMaxSize=off  VariableDim=1 (Row)  MaxSize=[1 1]  TunabilityNumber=1  MinValue=MinValue  MaxValue=MaxValue  TriggerInit=[20 25 190 75]  MaskValue=MaskValue
      settings: SourceProductName=Bose Talaria
  wires:
  Tune Variable/1 -> TrivialTranslation/1  "Scale"
  TrivialTranslation/1 -> TOP/1

== system Model_TranslationEngine64/NEAR/Near1p1/DrProc/FsEQDr ==
  note: FsEQArray
  note: The function-call generator block is temporarily added to allow code gen
  Pooliir : Subsystem  mask(Bose Pool IIR Tunable){FeatureName=Pooliir, Config=Config.Pooliir}
      mask prompts: FeatureName "Filter name/purpose"; Config "PoolIirTunableConfig"
      mask help:
      | Pool IIR Tunable is a configurable multi-channel IIR filter that supports one or more channels. This block offers flexibility of tuning the number of stages and coefficients. Different filter coefficients and number of stages (biquads) can be used for each channel filter. The Pool IIR Tunable block supports different implementations, which could be configured at build-time:
      |
      | (i)   Generic: IIR filter code not optimized for any processor
      | (ii)  SharcCore: IIR filters executing on core (uses pooliir.asm CRL)
      | (iii) SharcGulAccel: IIR filters executing on IIR hardware accelerator, offloading MIPS usage from core
      | (iv) SharcGxpAccel: IIR filters take advantage of additional accelerators available on GXP processor
      | (v)  Hexagon: TBD
      |
      | NOTE: When using Pool IIR for Sharc-plus based processors, the codeWorkMemory buffer and input buffer should always be mapped to L1 memory to optimize MIPS utilization and avoid audio artifacts.
      |
      | For more information, please see 'Help'.
      mask init:
      | blkh=gcbh;
      | Config=BTConfig.Assert(blkh,Config);
      | 
      | Config.Validate();
      | Config.DoMaskInit(blkh);
      mask Help:
      | <b>Input signals: </b>
      | AudioIn: input channels [frame size x number of channels]
      | 
      | <b>Output signals: </b>
      | AudioOut: output channels [frame size x number of channels]
      | 
      | <b>Mask parameters: </b>
      | PoolIirTunableConfig
      | Filter name/purpose
      mask TypeOptions FeatureName: PoolIirTunableWithReset/FeatureName
      mask Display: DrawPoolIirIcon;
  Subsystem1 : Subsystem

== system Model_TranslationEngine64/NEAR/Near1p1/DrProc/HrEQDr ==
  note: The function-call generator block is temporarily added to allow code gen
  PoolIirTunable : Subsystem  mask(Bose Pool IIR Tunable){FeatureName=PoolIirTunable, Config=Config.PoolIirTunable}
      mask prompts: FeatureName "Filter name/purpose"; Config "PoolIirTunableConfig"
      mask help:
      | Pool IIR Tunable is a configurable multi-channel IIR filter that supports one or more channels. This block offers flexibility of tuning the number of stages and coefficients. Different filter coefficients and number of stages (biquads) can be used for each channel filter. The Pool IIR Tunable block supports different implementations, which could be configured at build-time:
      |
      | (i)   Generic: IIR filter code not optimized for any processor
      | (ii)  SharcCore: IIR filters executing on core (uses pooliir.asm CRL)
      | (iii) SharcGulAccel: IIR filters executing on IIR hardware accelerator, offloading MIPS usage from core
      | (iv) SharcGxpAccel: IIR filters take advantage of additional accelerators available on GXP processor
      | (v)  Hexagon: TBD
      |
      | NOTE: When using Pool IIR for Sharc-plus based processors, the codeWorkMemory buffer and input buffer should always be mapped to L1 memory to optimize MIPS utilization and avoid audio artifacts.
      |
      | For more information, please see 'Help'.
      mask init:
      | blkh=gcbh;
      | Config=BTConfig.Assert(blkh,Config);
      | 
      | Config.Validate();
      | Config.DoMaskInit(blkh);
      mask Help:
      | <b>Input signals: </b>
      | AudioIn: input channels [frame size x number of channels]
      | 
      | <b>Output signals: </b>
      | AudioOut: output channels [frame size x number of channels]
      | 
      | <b>Mask parameters: </b>
      | PoolIirTunableConfig
      | Filter name/purpose
      mask TypeOptions FeatureName: PoolIirTunableWithReset/FeatureName
      mask Display: DrawPoolIirIcon;
  Subsystem2 : Subsystem

== system Model_TranslationEngine64/NEAR/Near1p1/DrProc/RouterDr ==
  InnerLink : Subsystem  mask(Blocklib Router){Config=InnerLinkConfig, FeatureName=Router}
      mask prompts: Config "RouterConfig"; FeatureName "Feature path name:"
      mask help: This block allows the user to route X input channels to Y output channels. Enter a value of 0 to "zero out" the specific channel
      mask init:
      | blkh=gcbh;
      | Config=BTConfig.Assert(blkh,Config);
      | 
      | Config.Validate();
      | BTConfig.InitSetFeatureIfPresent(blkh,'FeatureName');
      mask Callback Config: BTConfig.CallbackHideIfPresent(gcbh,{'FeatureName'});
      mask TypeOptions FeatureName: FeaturePath/FeatureName
      mask Display: image('routerIcon.png');

== system Model_TranslationEngine64/NEAR/Near1p1/DrProc/Upmixer1p1Dr ==
  Subsystem1 : Subsystem

== system Model_TranslationEngine64/NEAR/Near1p1/FrProc/Subsystem ==
  FeaturePath : FeaturePath/FeaturePath  FeatureName=Fr_  IsGroup=off  GroupNumber=-1  IsModule=off  TriggerInit=[760 79 875 186]
      settings: SourceProductName=Bose Talaria
  FsEQFr : Subsystem  mask(FsEQ){Config=Config.FsEqFr}
      mask prompts: Config "FsEqConfig"
      mask help:
      | This mask allows the setting of parameters for the FsEQ model.
      | Model parameters are set by a class instance in the base workspace.
      |
      | See 'Help' for details.
      mask init:
      | blkh=gcbh;
      | Config=BTConfig.Assert(blkh,Config);
      | 
      | Config.Validate();
      | Config.DoMaskInit(blkh);
      mask Help:
      | Defining model parameters:
      | The model parameters are set by the conents of an instance of FsEQClass.m.
      | 
      | To set model parameters:
      | 1-Create an instance of FsEQClass.m in the base workspace.
      | 2-In the model mask, set the 'Class instance' parameter to the name of the class instance in the base workspace.
      mask DialogControl ClassContainer Prompt: Name of class instance containing parameter settings
  HrEQFr : Subsystem  mask(HrEQ){Config=Config.HrEqFr}
      mask prompts: Config "HrEqConfig"
      mask help:
      | This mask allows the setting of parameters for the HrEQ model.
      | Model parameters are set by a class instance in the base workspace.
      |
      | See 'Help' for details.
      mask init:
      | blkh=gcbh;
      | Config=BTConfig.Assert(blkh,Config);
      | 
      | Config.Validate();
      | Config.DoMaskInit(blkh);
      mask Help:
      | Defining model parameters:
      | The model parameters are set by the conents of an instance of HrEQClass.m.
      | 
      | To set model parameters:
      | 1-Create an instance of HrEQClass.m in the base workspace.
      | 2-In the model mask, set the 'Class instance' parameter to the name of the class instance in the base workspace.
  RouterFr : Subsystem  mask(Bose Router){nInRouterMask=Config.NearRouterNumIn, nOutRouterMask=Config.NearRouterNumOut, outputMapDefaultRouterMask=Config.NearRouterMap}
      mask prompts: nInRouterMask "Number of input channels"; nOutRouterMask "Number of output channels"; outputMapDefaultRouterMask "Router output channel indices"
      mask help: This block allows the user to route X input channels to Y output channels. Enter a value of 0 to "zero out" the specific channel
      mask init: same as Model_TranslationEngine64/NEAR/Near1p1/DrProc/RouterDr
      mask Display: image('routerIcon.png');
  Upmixer1p1Fr : Subsystem  mask{Config=Config.Upmixer1p1Fr}
      mask prompts: Config "Upmixer1p1Config"
      mask init: same as Model_TranslationEngine64/NEAR/Near1p1/DrProc/Upmixer1p1Dr

== system Model_TranslationEngine64/NEAR/Near1p1/LocRamper/TuneTOP ==
  TOP : TOP/TOP  TriggerInit=[440 20 585 80]  TopName=RampDbPerSample  DataTypeOut=single  BankNumber=BankNumber  PreOverlay=PreOverlay  PostOverlay=PostOverlay  Role=Automatic
      settings: SourceProductName=Bose Talaria
  TrivialTranslation : TuneVar/TrivialTranslation  TriggerInit=[300 28 350 72]
      settings: SourceProductName=Bose Talaria
  Tune Variable : TuneVar/TuneVar  TuneName=RampDbPerSample  SpecifyMaxSize=off  VariableDim=1 (Row)  MaxSize=[1 1]  TunabilityNumber=1  MinValue=MinValue  MaxValue=MaxValue  TriggerInit=[20 25 190 75]  MaskValue=MaskValue
      settings: SourceProductName=Bose Talaria
  wires:
  Tune Variable/1 -> TrivialTranslation/1  "RampDbPerSample"
  TrivialTranslation/1 -> TOP/1

== system Model_TranslationEngine64/NEAR/Near1p1/NearBandSplit/HighpassFilter ==
  note: The function-call generator block is temporarily added to allow code gen
  HpfCutOffTuneVar : TuneVar/TuneVar  TuneName=HpfCutoffFrequency  SpecifyMaxSize=off  VariableDim=1 (Row)  MaxSize=[1 1]  TunabilityNumber=1  MinValue=[]  MaxValue=[]  TriggerInit=[25 295 195 345]  MaskValue=Config.DefaultHpfCutoffFrequency
      settings: SourceProductName=Bose Talaria
  HpfOrderTuneVar : TuneVar/TuneVar  TuneName=HpfFilterOrder  SpecifyMaxSize=off  VariableDim=1 (Row)  MaxSize=[1 1]  TunabilityNumber=1  MinValue=[]  MaxValue=[]  TriggerInit=[25 375 195 425]  MaskValue=Config.DefaultHpfFilterOrder
      settings: SourceProductName=Bose Talaria
  NumChannelsCapConst : CapturedConstLib/CapturedConst  TriggerInit=[85 542 185 578]  Role=Automatic
      settings: SourceProductName=Bose Talaria
  SampleRateCapConst : CapturedConstLib/CapturedConst  TriggerInit=[85 462 185 498]  Role=Automatic
      settings: SourceProductName=Bose Talaria
  TOP : TOP/TOP  TriggerInit=[740 1240 885 1300]  TopName=Coefficients  DataTypeOut=single  BankNumber=0  PreOverlay=false  PostOverlay=false  Role=Automatic
      settings: SourceProductName=Bose Talaria
  TOP1 : TOP/TOP  TriggerInit=[740 1080 885 1140]  TopName=NumStages  DataTypeOut=uint32  BankNumber=0  PreOverlay=false  PostOverlay=false  Role=Automatic
      settings: SourceProductName=Bose Talaria
  TranslateTrigger : TuneVar/TranslateTrigger  TriggerInit=[591 950 629 1005]
      settings: SourceProductName=Bose Talaria
  Translation : MATLAB Function  TreatAsAtomicUnit=on
  wires:
  SampleRateCapConst/1 -> Translation/3(sampleRate)
  HpfOrderTuneVar/1 -> Translation/2(order)  "HpfFilterOrder"
  TranslateTrigger/1 -> Translation/Trigger
  Translation/2(LRHighPassCoeffs) -> TOP/1
  NumChannelsCapConst/1 -> Translation/4(numChannels)
  HpfCutOffTuneVar/1 -> Translation/1(crossOverFrequency)  "HpfCutoffFrequency"
  Translation/1(LRHighPassNumStages) -> TOP1/1

== system Model_TranslationEngine64/NEAR/Near1p1/VolumeMute/AnnouncementLevelDetector ==
  PreProcessing : Subsystem
  ch1_level : Subsystem
  ch2_level : Subsystem
  ch3_level : Subsystem
  ch4_level : Subsystem
